simulink model "PandO"  (R2020a)
settings: Solver=VariableStepAuto  StartTime=0.0  StopTime=10.0  RelTol=1e-3
libraries: powerlib_meascontrol x1
settings Model: Creator=sameeraa  LastModifiedBy=sameeraa

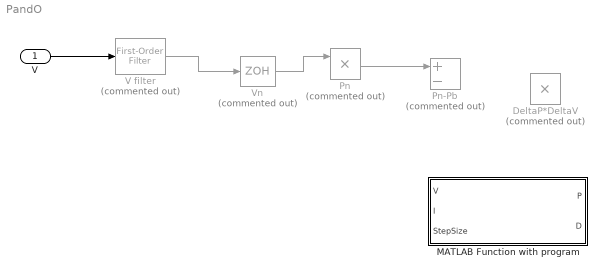
== system PandO ==
  V : Inport
  DeltaP*DeltaV : Product  Commented=on
  MATLAB Function with program : MATLAB Function  TreatAsAtomicUnit=on
  Pn : Product  Commented=on
  Pn-Pb : Sum  Commented=on  Inputs=+-
  V filter : powerlib_meascontrol/Filters/First-Order Filter  Commented=on  FilterType=Lowpass  Tc=10e-3  Ts=0  Initialize=on  Vac_Init=[0, 0, 60]  Vdc_Init=0  PlotResponse=off  FreqRange="[0,  200,  1]"
  Vn : ZeroOrderHold  Commented=on  SampleTime=-1
  wires:
  V/1 -> V filter/1
  V filter/1 -> Vn/1
  Vn/1 -> Pn/1
  Pn/1 -> Pn-Pb/1

== matlab function PandO/MATLAB Function with program ==
  data: V input; P output; I input; StepSize input; D output
function [P, D] = fcn(V,I,StepSize)
    % Initialization
    persistent Pprev Vprev Dprev
    if isempty(Pprev)
        Pprev = 0;
        Vprev = 0;
        Dprev = 0.5;
    end
    % P&O Algorithm Begin here
    P = I*V;
    if (P-Pprev) > 0
        if (V-Vprev) > 0
            D = Dprev - StepSize;
        else
            D = Dprev + StepSize;
        end
    else
        if (V-Vprev) > 0
            D = Dprev + StepSize;
        else
            D = Dprev - StepSize;
        end
    end
    % Update current value to previous value
    Pprev = P;
    Vprev = V;
    Dprev = D;
end
